simulink model "motor_model"  (R2015a)
settings: Solver=ode1  StartTime=0.0  StopTime=inf  FixedStep=0.002  RelTol=1e-3
undefined symbols (not defined in the file): HIL, Jeq, km, kt, Rm
libraries: quarc_library x4, simulink x3, simulink_extras x3
settings Model: SimulationMode=external  ExtModeTrigDuration=10000  Creator=bemran  LastModifiedBy=bemran
settings SolverCC: PositivePriorityOrder=on
settings DataIOCC: LimitDataPoints=off
settings RTWCC: SystemTargetFile=quarc_win64.tlc  TemplateMakefile=quarc_default_tmf  Description=QUARC Win64 Target
settings STFCustomTargetCC: TargetLibSuffix=.lib  TargetPreCompLibLocation=C:\PROGRA~3\QUARC\lib\2015a\win64\release  GenerateSampleERTMain=off  ConcurrentExecutionCompliant=on  GeneratePreprocessorConditionals=Disable all  ERTCustomFileBanners=off  SupportNonInlinedSFcns=on  SupportVariableSizeSignals=off  MATLABClassNameForMDSCustomization=Simulink.SoftwareTarget.GRTCustomization  GRTInterface=on  SystemTargetFile=quarc_win64.tlc
settings GRTTargetCC: TargetPreCompLibLocation=C:\PROGRA~3\QUARC\lib\2015a\win64\release  ParMdlRefBuildCompliant=off  CompOptLevelCompliant=off  CombineOutputUpdateFcns=off  MatFileLogging=off  CPPClassGenCompliant=off  GRTInterface=on  ExtMode=on  ExtModeMexFile=quarc_comm

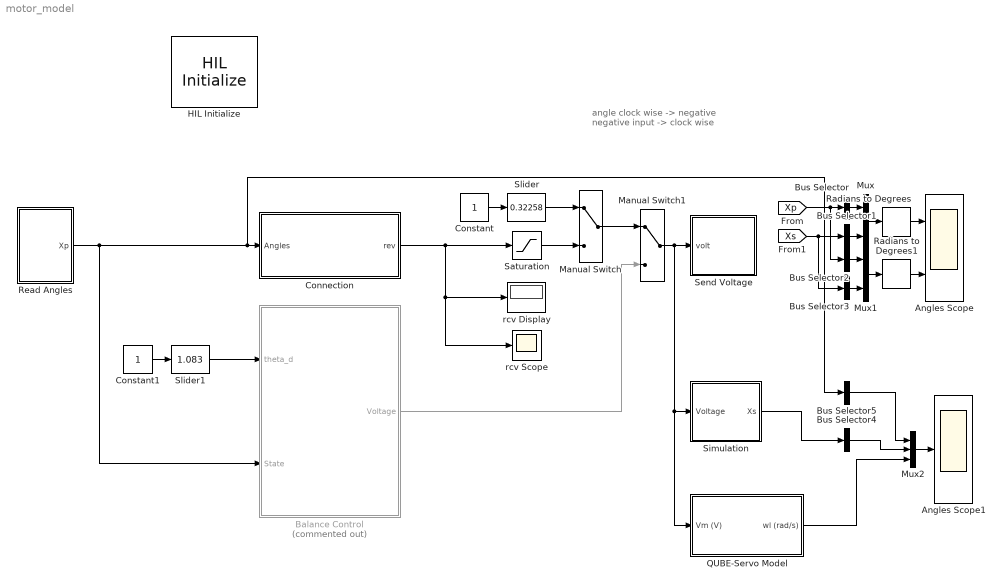
== system motor_model ==
  note: angle clock wise -> negative
      | negative input -> clock wise
  Angles Scope : Scope  NumInputPorts=2
      settings: YMin=-45000~-2750  YMax=0~0  SaveName=ScopeData2
  Angles Scope1 : Scope
      settings: YMin=-50  YMax=50
  Balance Control : Subsystem  Commented=on
  Bus Selector{,1,3..4} (4 alike) : BusSelector  OutputSignals=theta  OutputAsBus=on
  Bus Selector2 : BusSelector  OutputSignals=w  OutputAsBus=on
  Bus Selector5 : BusSelector  OutputSignals=w  OutputAsBus=on
  Connection : Subsystem  Variant=on  OverrideUsingVariant=tcp_connection
  Constant : Constant
  Constant1 : Constant
  HIL Initialize : quarc_library/Data Acquisition/Generic/Configuration/HIL Initialize  Priority=-99  object_name=HIL-1  board_type=qube_servo2_usb  board_number=0  board_options=""  exclusive=off  active=off  hardware_clocks=[0]  clock_modes=[]  initial_clock_frequencies=[]  set_clock_params_at_start=off  set_clock_params_at_switch_in=off  set_clock_frequencies_at_start=off  set_clock_frequencies_at_switch_in=off  analog_input_channels=[0]  analog_input_maximums=3  analog_input_minimums=-3  set_analog_input_params_at_start=off  set_analog_input_params_at_switch_in=off  analog_output_channels=[0]  analog_output_maximums=15  analog_output_minimums=-15  initial_analog_outputs=[0]  final_analog_outputs=[0]  watchdog_analog_outputs=0  set_analog_output_params_at_start=off  set_analog_output_params_at_switch_in=off  set_analog_outputs_at_start=on  set_analog_outputs_at_switch_in=off  set_analog_outputs_at_terminate=on  set_analog_outputs_at_switch_out=off  set_analog_outputs_on_watchdog=on  digital_input_channels=[]  digital_output_channels=[0]  digital_output_configuration=[]  initial_digital_outputs=[1]  final_digital_outputs=[0]  watchdog_digital_outputs=[0]  set_digital_output_params_at_start=off  set_digital_output_params_at_switch_in=off  set_digital_outputs_at_start=on  set_digital_outputs_at_switch_in=off  set_digital_outputs_at_terminate=on  set_digital_outputs_at_switch_out=off  set_digital_outputs_on_watchdog=on  encoder_channels=[0:1]  quadrature=[4]  encoder_filter_frequency=[]  initial_encoder_counts=[0]  set_encoder_params_at_start=off  set_encoder_params_at_switch_in=off  set_encoder_counts_at_start=on  set_encoder_counts_at_switch_in=off  pwm_channels=[]  pwm_modes=[]  pwm_frequency=[]  pwm_configuration=[]  pwm_alignment=[]  pwm_polarity=[]  pwm_leading_deadband=[]  pwm_trailing_deadband=[]  initial_pwm_outputs=[]  final_pwm_outputs=[]  watchdog_pwm_outputs=[]  set_pwm_params_at_start=off  set_pwm_params_at_switch_in=off  set_pwm_outputs_at_start=off  set_pwm_outputs_at_switch_in=off  set_pwm_outputs_at_terminate=off  set_pwm_outputs_at_switch_out=off  set_pwm_outputs_on_watchdog=off  other_output_channels=[11000:11002]  initial_other_outputs=[0 1 0]  final_other_outputs=[1 0 0]  watchdog_other_outputs=[0 0 1]  set_other_outputs_at_start=on  set_other_outputs_at_switch_in=off  set_other_outputs_at_terminate=on  set_other_outputs_at_switch_out=off  set_other_outputs_on_watchdog=on
  Manual Switch : ManualSwitch
  Manual Switch1 : ManualSwitch
  Mux : Mux  Inputs=2
  Mux1 : Mux  Inputs=2
  Mux2 : Mux  Inputs=3
  QUBE-Servo Model : Subsystem
  Radians to Degrees : simulink_extras/Transformations/Radians to Degrees
  Radians to Degrees1 : simulink_extras/Transformations/Radians to Degrees
  Read Angles : Subsystem
  Saturation : Saturate  UpperLimit=5  LowerLimit=-5
  Send Voltage : Subsystem
  Simulation : Subsystem
  Slider : simulink/Math Operations/Slider Gain  low=0  gain=0.32258  high=5
  Slider1 : simulink/Math Operations/Slider Gain  low=0  gain=1.083  high=5
  rcv Display : Display
  rcv Scope : Scope
  wires:
  Constant/1 -> Slider/1
  Mux/1 -> Radians to Degrees/1
  Radians to Degrees/1 -> Angles Scope/1
  Connection/1(rev) -> Saturation/1, rcv Scope/1, rcv Display/1
  Read Angles/1(Xp) -> Balance Control/2("State "), Bus Selector5/1, Connection/1(Angles)
  Radians to Degrees1/1 -> Angles Scope/2
  [Xp] -> Bus Selector2/1, Bus Selector/1
  Slider/1 -> Manual Switch/1
  Manual Switch/1 -> Manual Switch1/1
  Saturation/1 -> Manual Switch/2
  Constant1/1 -> Slider1/1
  Slider1/1 -> Balance Control/1(theta_d)
  Balance Control/1(Voltage) -> Manual Switch1/2
  Manual Switch1/1 -> QUBE-Servo Model/1(Vm (V)), Simulation/1(Voltage), Send Voltage/1(volt)
  Bus Selector/1 -> Mux/1
  Mux1/1 -> Radians to Degrees1/1
  Bus Selector2/1 -> Mux1/1
  [Xs] -> Bus Selector3/1, Bus Selector1/1
  Bus Selector3/1 -> Mux1/2
  Bus Selector1/1 -> Mux/2
  Mux2/1 -> Angles Scope1/1
  QUBE-Servo Model/1(wl (rad/s)) -> Mux2/3
  Simulation/1(Xs) -> Bus Selector4/1
  Bus Selector4/1 -> Mux2/2
  Bus Selector5/1 -> Mux2/1

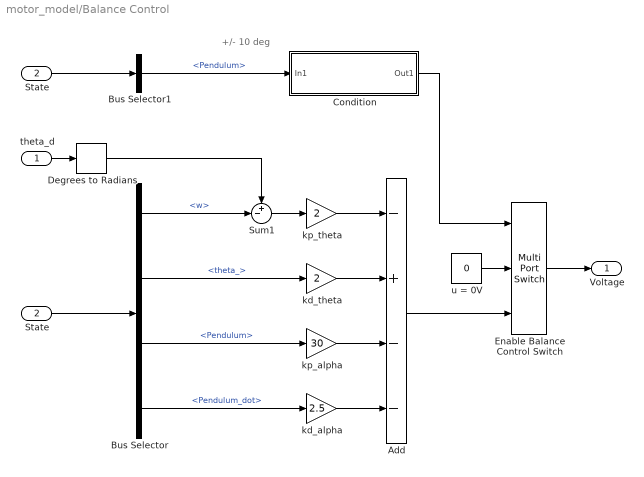
== system motor_model/Balance Control ==
  note: +/- 10 deg
  theta_d : Inport
  "State " : Inport  Port=2
  Add : Sum  Inputs=-+--
  Bus Selector : BusSelector  OutputSignals=w,theta_,Pendulum,Pendulum_dot
  Bus Selector1 : BusSelector  OutputSignals=Pendulum
  Condition : Subsystem
  Degrees to Radians : simulink_extras/Transformations/Degrees to Radians
  Enable Balance Control Switch : MultiPortSwitch  DataPortOrder=Zero-based contiguous  Inputs=2  zeroidx=on
  State : InportShadow  Port=2
  Sum1 : Sum  Inputs=+-|
  kd_alpha : Gain  Gain=2.5
  kd_theta : Gain  Gain=2
  kp_alpha : Gain  Gain=30
  kp_theta : Gain  Gain=2
  u = 0V : Constant  Value=0
  Voltage : Outport
  wires:
  u = 0V/1 -> Enable Balance Control Switch/2
  Bus Selector/4 -> kd_alpha/1  "<Pendulum_dot>"
  Bus Selector/2 -> kd_theta/1  "<theta_>"
  kp_theta/1 -> Add/1
  kd_theta/1 -> Add/2
  kp_alpha/1 -> Add/3
  kd_alpha/1 -> Add/4
  Add/1 -> Enable Balance Control Switch/3
  Enable Balance Control Switch/1 -> Voltage/1
  Sum1/1 -> kp_theta/1
  theta_d/1 -> Degrees to Radians/1
  Degrees to Radians/1 -> Sum1/1
  Condition/1(Out1) -> Enable Balance Control Switch/1
  "State "/1 -> Bus Selector/1
  Bus Selector/1 -> Sum1/2  "<w>"
  State/1 -> Bus Selector1/1
  Bus Selector1/1 -> Condition/1(In1)  "<Pendulum>"
  Bus Selector/3 -> kp_alpha/1  "<Pendulum>"

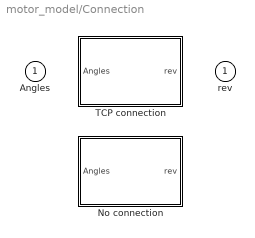
== system motor_model/Connection ==
  Angles : Inport
  No connection : Subsystem  VariantControl=no_connection
  TCP connection : Subsystem  VariantControl=tcp_connection
  rev : Outport

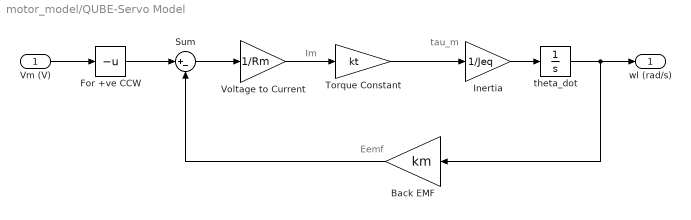
== system motor_model/QUBE-Servo Model ==
  note: Im
  note: tau_m
  note: Eemf
  Vm (V) : Inport
  Back EMF : Gain  Gain=km  SaturateOnIntegerOverflow=on  OutDataTypeStr=Inherit: Same as input  ParamDataTypeStr=Inherit: Same as input
  For +ve CCW : UnaryMinus
  Inertia : Gain  Gain=1/Jeq  SaturateOnIntegerOverflow=on  OutDataTypeStr=Inherit: Same as input  ParamDataTypeStr=Inherit: Same as input
  Sum : Sum  Inputs=|+-  SaturateOnIntegerOverflow=on  InputSameDT=on  OutDataTypeStr=Inherit: Same as first input
  Torque Constant : Gain  Gain=kt
  Voltage to Current : Gain  Gain=1/Rm  SaturateOnIntegerOverflow=on  OutDataTypeStr=Inherit: Same as input  ParamDataTypeStr=Inherit: Same as input
  theta_dot : Integrator
  wl (rad/s) : Outport
  wires:
  Voltage to Current/1 -> Torque Constant/1
  Vm (V)/1 -> For +ve CCW/1
  Sum/1 -> Voltage to Current/1
  theta_dot/1 -> Back EMF/1, wl (rad/s)/1
  Torque Constant/1 -> Inertia/1
  Inertia/1 -> theta_dot/1
  Back EMF/1 -> Sum/2
  For +ve CCW/1 -> Sum/1

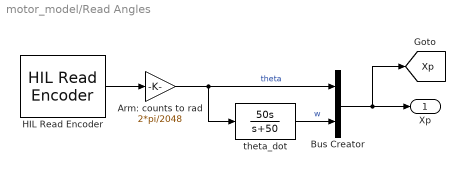
== system motor_model/Read Angles ==
  Arm: counts to rad : Gain  Gain=2*pi/2048
  Bus Creator : BusCreator  Inputs=2
  HIL Read Encoder : quarc_library/Data Acquisition/Generic/Immediate I//O/HIL Read Encoder  object_name=HIL-1  channels=0  sample_time=qc_get_step_size  active=on  vector_output=off  data_type_mode=Inherit via back propagation  data_type=double
  theta_dot : TransferFcn  Numerator=[50 0]  Denominator=[1 50]
  Xp : Outport
  tag scope: Xp=global
  wires:
  Arm: counts to rad/1 -> theta_dot/1, Bus Creator/1  "theta"
  HIL Read Encoder/1 -> Arm: counts to rad/1
  Bus Creator/1 -> Xp/1, [Xp]
  theta_dot/1 -> Bus Creator/2  "w"

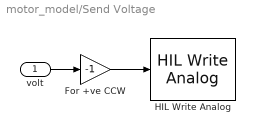
== system motor_model/Send Voltage ==
  volt : Inport
  For +ve CCW : Gain  Gain=-1
  HIL Write Analog : quarc_library/Data Acquisition/Generic/Immediate I//O/HIL Write Analog  object_name=HIL-1  channels=0  sample_time=-1  active=off  vector_input=off
  wires:
  volt/1 -> For +ve CCW/1
  For +ve CCW/1 -> HIL Write Analog/1

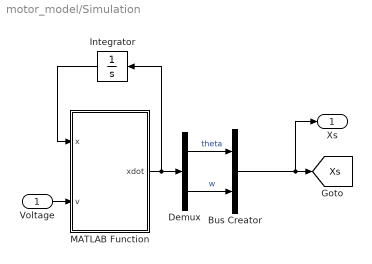
== system motor_model/Simulation ==
  Voltage : Inport
  Bus Creator : BusCreator  Inputs=2
  Demux : Demux  Outputs=2
  Integrator : Integrator  InitialCondition=[0,0]
  MATLAB Function : MATLAB Function  TreatAsAtomicUnit=on
  Xs : Outport
  tag scope: Xs=global
  wires:
  Integrator/1 -> MATLAB Function/1(x)
  Voltage/1 -> MATLAB Function/2(v)
  MATLAB Function/1(xdot) -> Demux/1, Integrator/1
  Demux/1 -> Bus Creator/1  "theta"
  Demux/2 -> Bus Creator/2  "w"
  Bus Creator/1 -> [Xs], Xs/1

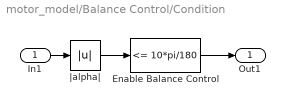
== system motor_model/Balance Control/Condition ==
  In1 : Inport
  Enable Balance Control : simulink/Logic and Bit Operations/Compare To Constant  relop=<=  const=10*pi/180  OutDataTypeStr=uint8  ZeroCross=off
  |alpha| : Abs
  Out1 : Outport
  wires:
  |alpha|/1 -> Enable Balance Control/1
  Enable Balance Control/1 -> Out1/1
  In1/1 -> |alpha|/1

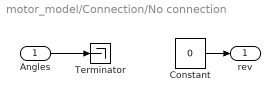
== system motor_model/Connection/No connection ==
  Angles : Inport
  Constant : Constant  Value=0
  Terminator : Terminator
  rev : Outport
  wires:
  Constant/1 -> rev/1
  Angles/1 -> Terminator/1

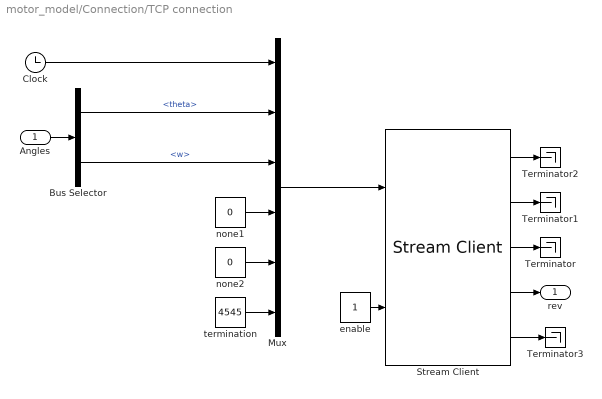
== system motor_model/Connection/TCP connection ==
  Angles : Inport
  Bus Selector : BusSelector  OutputSignals=theta,w
  Clock : Clock
  Mux : Mux  Inputs=6
  Stream Client : quarc_library/Communications/Basic/Stream Client  uri_source=Specify via dialog (do not evaluate)  uri=tcpip://127.0.0.1:18001  apply_uri_to_all_configs=on  send_buffer_size=1460  receive_buffer_size=1460  byte_order=big endian (Motorola - MSB first)  optimization=Minimum latency  implementation=Use blocking I/O in a separate thread  send_options=Send most recent data  receive_options=Receive most recent data  send_fifo_size=1000  receive_fifo_size=1000  send_priority=0  receive_priority=0  default_value=[0]  send_dimensions=off  receive_dimensions=off  max_dimensions=-1  sample_time=qc_get_step_size  active=off  data_type=Inherited via back propagation  type_expr=BusObject
      settings: AttributesFormatString="\"tcpip://127.0.0.1:18001\""
  Terminator{,1..3} (4 alike) : Terminator
  enable : Constant
  none1 : Constant  Value=0
  none2 : Constant  Value=0
  termination : Constant  Value=4545
  rev : Outport
  wires:
  Stream Client/5 -> Terminator3/1
  Angles/1 -> Bus Selector/1
  Stream Client/4 -> rev/1
  enable/1 -> Stream Client/2
  Clock/1 -> Mux/1
  Stream Client/1 -> Terminator2/1
  Stream Client/2 -> Terminator1/1
  Stream Client/3 -> Terminator/1
  Mux/1 -> Stream Client/1
  termination/1 -> Mux/6
  Bus Selector/1 -> Mux/2  "<theta>"
  Bus Selector/2 -> Mux/3  "<w>"
  none1/1 -> Mux/4
  none2/1 -> Mux/5

== matlab function motor_model/Simulation/MATLAB Function ==
  data: x input; v input; xdot output
function xdot  = dynamics (x, v)

Rm = 8.4;           % Resistance
kt = 0.042;         % Current-torque (N-m/A)
km = 0.042;         % Back-emf constant (V-s/rad)
Jr = 4e-6;          % Rotor inertia (kg-m^2)
mh = 0.0106;        % 9 g Hub mass (kg)
rh = 22.2/1000/2;   % Hub radius (m) diameter 22.2 mm
Jh = 0.5*mh*rh^2;   % Hub inertia (kg-m^2)
md = 0.053;         % Disc mass (kg)
rd = 49.5/1000/2;   % Disc radius (m) diameter = 49.5 mm
Jd = 0.5*md*rd^2;   % Disc moment of inertia (kg-m^2)
Jeq = Jr + Jh + Jd; % Equivalent moment of inertia (kg-m^2)

theta = x(1);
w = x(2);

theta_dot = w;
w_dot = kt * (-v - km * w) / Rm /Jeq;

xdot = [theta_dot, w_dot];
